simulink model "auv5dof"  (R2021a)
settings: Solver=VariableStepAuto  StartTime=0.0  StopTime=300.00  RelTol=1e-3
settings Model: Creator=aditya-ubuntu  LastModifiedBy=mluser
settings SolverCC: AlgebraicLoopSolver=TrustRegion
settings DataIOCC: ReturnWorkspaceOutputs=off
settings DebuggingCC: SFMachineParentedDataDiag=warning  ArithmeticOperatorsInVariantConditions=warning
settings SFSimCC: CustomCodeUndefinedFunction=UseInterfaceOnly

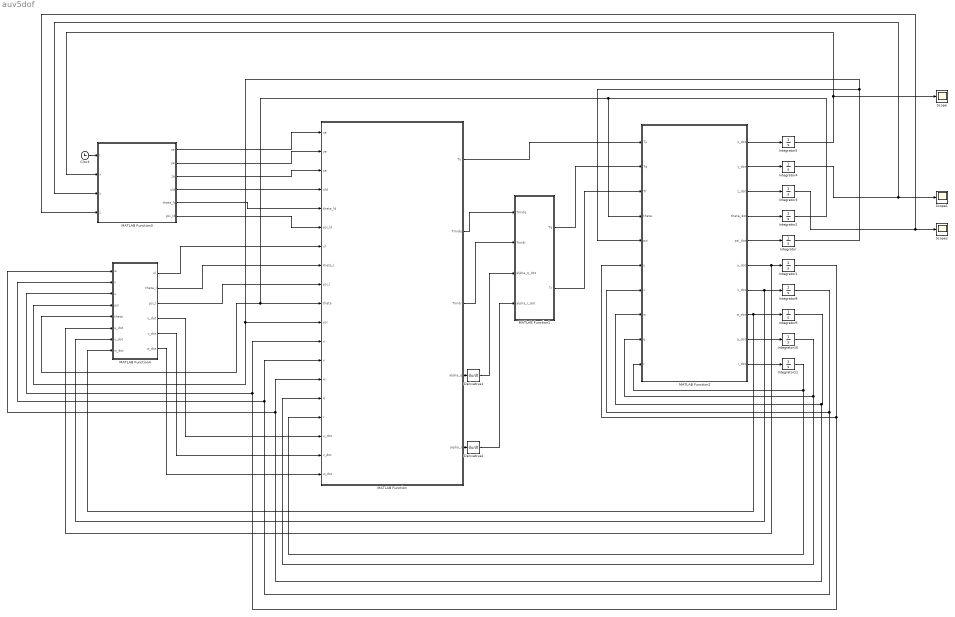
== system auv5dof ==
  Clock : Clock
  Derivative1 : Derivative
  Derivative2 : Derivative
  Integrator{,1..5,8..11} (10 alike) : Integrator
  MATLAB Function : MATLAB Function  TreatAsAtomicUnit=on
  MATLAB Function1 : MATLAB Function  TreatAsAtomicUnit=on
  MATLAB Function2 : MATLAB Function  TreatAsAtomicUnit=on
  MATLAB Function3 : MATLAB Function  TreatAsAtomicUnit=on
  MATLAB Function4 : MATLAB Function  TreatAsAtomicUnit=on
  Scope : Scope
  Scope1 : Scope
  Scope2 : Scope
  wires:
  MATLAB Function2/1(x_dot) -> Integrator5/1
  MATLAB Function2/2(y_dot) -> Integrator4/1
  MATLAB Function2/3(z_dot) -> Integrator3/1
  MATLAB Function2/4(theta_dot) -> Integrator2/1
  MATLAB Function2/5(psi_dot) -> Integrator/1
  MATLAB Function2/6(u_dot) -> MATLAB Function4/6("u_dot "), Integrator1/1
  Integrator5/1 -> Scope/1, MATLAB Function3/2(x)
  Integrator4/1 -> MATLAB Function3/3(y), Scope1/1
  MATLAB Function2/7(v_dot) -> MATLAB Function4/7("v_dot "), Integrator8/1
  MATLAB Function2/8(w_dot) -> MATLAB Function4/8("w_dot "), Integrator9/1
  MATLAB Function2/9(q_dot) -> Integrator10/1
  MATLAB Function2/10(r_dot) -> Integrator11/1
  Integrator10/1 -> MATLAB Function/15(q), MATLAB Function2/9(q)
  Integrator9/1 -> MATLAB Function4/1(w), MATLAB Function/14(w), MATLAB Function2/8(w)
  Integrator8/1 -> MATLAB Function/13(v), MATLAB Function4/2(v), MATLAB Function2/7(v)
  Integrator1/1 -> MATLAB Function/12(u), MATLAB Function4/3(u), MATLAB Function2/6(u)
  Integrator/1 -> MATLAB Function2/5(psi), MATLAB Function4/4(psi), MATLAB Function/11(psi)
  Integrator2/1 -> MATLAB Function4/5(theta), MATLAB Function/10(theta), MATLAB Function2/4(theta)
  Integrator11/1 -> MATLAB Function/16(r), MATLAB Function2/10(r)
  MATLAB Function4/2(theta_l) -> MATLAB Function/8(theta_l)
  MATLAB Function4/3(psi_l) -> MATLAB Function/9(psi_l)
  MATLAB Function4/1(ul) -> MATLAB Function/7(ul)
  MATLAB Function3/1(xe) -> MATLAB Function/1(xe)
  MATLAB Function3/2(ye) -> MATLAB Function/2(ye)
  MATLAB Function3/3(ze) -> MATLAB Function/3(ze)
  MATLAB Function3/4(uld) -> MATLAB Function/4(uld)
  MATLAB Function3/5(theta_ld) -> MATLAB Function/5(theta_ld)
  MATLAB Function3/6(psi_ld) -> MATLAB Function/6(psi_ld)
  Integrator3/1 -> MATLAB Function3/4(z), Scope2/1
  Clock/1 -> MATLAB Function3/1(t)
  MATLAB Function/1(Tu) -> MATLAB Function2/1(Tu)
  MATLAB Function/2(Tmidq) -> MATLAB Function1/1(Tmidq)
  MATLAB Function/3(Tmidr) -> MATLAB Function1/2(Tmidr)
  MATLAB Function/4(alpha_q) -> Derivative1/1
  Derivative1/1 -> MATLAB Function1/3(alpha_q_dot)
  MATLAB Function/5(alpha_r) -> Derivative2/1
  Derivative2/1 -> MATLAB Function1/4(alpha_r_dot)
  MATLAB Function1/1(Tq) -> MATLAB Function2/2(Tq)
  MATLAB Function1/2(Tr) -> MATLAB Function2/3(Tr)
  MATLAB Function4/4(u_dot) -> MATLAB Function/17(u_dot)
  MATLAB Function4/5(v_dot) -> MATLAB Function/18(v_dot)
  MATLAB Function4/6(w_dot) -> MATLAB Function/19(w_dot)

== matlab function auv5dof/MATLAB Function2 ==
  data: x_dot output; y_dot output; z_dot output; theta_dot output; psi_dot output; u_dot output; v_dot output; w_dot output; q_dot output; r_dot output; Tu input; Tq input; Tr input; theta input; psi input; u input; v input; w input; q input; r input
function [ x_dot, y_dot, z_dot, theta_dot, psi_dot, u_dot, v_dot, w_dot, q_dot, r_dot] = outputfn5dof(Tu, Tq, Tr, theta, psi, u, v, w, q, r)
    

    m = [ 1116 2133 2133 36.7 4061 4061];

    onebym = [1/1116 1/2133 1/2133 1/36.7 1/4061 1/4061];
    
    d = [ 25.5 138 138 10 490 490];
    
    row = 1000;
    g = 9.8;
    invtri = 1;
    Gml = 1;
    fu = (m(2)*v*r*onebym(1)) - (m(3)*w*q*onebym(1));
    fv = (-(m(1)*u*r*onebym(2)));
    fw = (m(1)*u*q*onebym(3));
    fq = ((m(3)-m(1))*u*w*onebym(5) - row*g*invtri*Gml*onebym(5)*sin(theta));
    fr = (m(1)-m(2))*u*v*onebym(6);
    
    x_dot = u*cos(theta)*cos(psi) - v*sin(psi) + w*sin(theta)*cos(psi);
    y_dot = u*cos(theta)*sin(psi) + v*cos(psi) + w*sin(theta)*sin(psi);
    z_dot = -u*sin(theta) + w*cos(theta);
    
    theta_dot = q;
    psi_dot = r*sec(theta);
    
    u_dot = fu- onebym(1)*Tu - d(1)*u*onebym(1);
    v_dot = fv - d(2)*onebym(2)*v;
    w_dot = fw - d(3)*onebym(3)*w;
    q_dot = fq + onebym(5)*Tq - d(5)*onebym(5)*q;
    r_dot = fr + onebym(6)*Tr - d(6)*onebym(6)*r; 
    
end

== matlab function auv5dof/MATLAB Function3 ==
  data: xe output; ye output; ze output; uld output; theta_ld output; psi_ld output; t input; x input; y input; z input
function [xe,ye,ze,uld,theta_ld,psi_ld] = fcn(t,x,y,z)
    
    if( t<= 90)
        xd = 0;
        yd = 0;
        zd = 0;
        uld = 1.5;
        theta_ld = 0;
        psi_ld = 0;
    else
        xd = 0;
        yd = 20;
        zd = 0;
        uld = 1.5;
        theta_ld = -10;
        psi_ld = 0.06;
    end
    
    xe = x - xd;
    ye = y - yd;
    ze = z - zd;
end

== matlab function auv5dof/MATLAB Function4 ==
  data: w input; v input; u input; psi input; theta input; ul output; theta_l output; psi_l output; u_dot output; v_dot output; w_dot output; u_dot input; v_dot input; w_dot input
function [ul, theta_l, psi_l, u_dot, v_dot, w_dot] = sphericalfcn(w,v,u,psi,theta, u_dot,v_dot,w_dot)
    
    ul = sqrt(u^2 + v^2 + w^2);
    theta_l = asin((sqrt(u^2+w^2)/ul)*(sin(theta + atan(-w/u))));
    psi_l = psi + atan(u/u*cos(theta));
    
end

== matlab function auv5dof/MATLAB Function1 ==
  data: Tq output; Tr output; Tmidq input; Tmidr input; alpha_q_dot input; alpha_r_dot input
function [Tq, Tr] = fcn(Tmidq, Tmidr, alpha_q_dot, alpha_r_dot)

    m5 = 4061;
    m6 = 4061;
    
    Tq = m5*( Tmidq + alpha_q_dot);
    Tr = m6*( Tmidr + alpha_r_dot);
       
end

== matlab function auv5dof/MATLAB Function ==
  data: Tu output; Tmidq output; Tmidr output; xe input; ye input; ze input; uld input; theta_ld input; psi_ld input; ul input; theta_l input; psi_l input; theta input; psi input; u input; v input; w input; q input; r input; alpha_q output; alpha_r output; u_dot input; v_dot input; w_dot input
function [Tu, Tmidq, Tmidr, alpha_q, alpha_r] = controlinputfn5dof(xe, ye, ze, uld, theta_ld, psi_ld, ul, theta_l, psi_l, theta, psi, u, v, w, q, r, u_dot, v_dot, w_dot)
    
    gamma_R = 0.2;
    gamma_r = 1.2;
    gamma_q = 1.2;
    gamma_u = 1;
    gamma_psi = 0.6;
    gamma_theta = 0.6;
    
    k_psi = 0.5;
    k_theta = 0.5;
    k_R = 0.01;
    k_u = 12;
    k_r = 0.9;
    k_q = 0.9;
    
    onebym_u = 1/1116;
    
    re = sqrt(xe^2 + ye^2 + ze^2);
    
    xe_dot = ul*cos(theta_l)*cos(psi_l) - uld*cos(theta_ld)*cos(psi_ld);
    ye_dot = ul*cos(theta_l)*sin(psi_l) - uld*cos(theta_ld)*sin(psi_ld);
    ze_dot = -ul*sin(theta_l) + uld*sin(theta_ld);
    
    theta_l_D_dot = ( (xe^2 + ye^2)*ze_dot - ze*( xe*xe_dot + ye*ye_dot)) / ( re^2*((xe^2 + ye^2)^0.5));
    psi_l_D_dot = ( xe*ye_dot - ye*xe_dot )/(xe^2+ye^2);
    theta_a = -atan(-w/sqrt(u^2+v^2));
    psi_a = atan(v/u);
    
    theta_b = atan( ze / sqrt(xe^2 + ye^2) );
    theta_le = theta_b - theta_l;
    alpha = theta + atan(-w/u);
    B = sqrt(u^2 + w^2)/ul;
    b_theta = (B*cos(alpha))/sqrt(1 - (B*sin(alpha)^2));
    B_dot = (u*u_dot + w*w_dot)/(ul*ul*B);
    
    F_theta_l = ( B_dot*sin(alpha) + B*cos(alpha)*(u_dot*w - u*w_dot)*(u^2 + w^2) ) / (sqrt(1- ((B*sin(alpha))^2)));
    alpha_q = b_theta^(-1)*( theta_l_D_dot - F_theta_l + (gamma_theta^(-1)*( k_theta*theta_le + ((sin(theta_le/2)^2)/(theta_le/2)))));
    eq = alpha_q - q;

    
    psi_b = atan2(ye,xe);
    psi_le = psi_b - psi_l;
    F_psi_l = ( (u*v_dot - u_dot*v)*cos(theta) + u*v*q*sin(theta) ) / ( (u*cos(theta)^2) + v^2 );
    alpha_r = cos(theta)*( psi_l_D_dot - F_psi_l + gamma_psi^(-1)*( k_psi*psi_le + ((sin(psi_le/2)^2)/(psi_le/2))));
    er = alpha_r - r;

    
    A = cos(theta_l)*cos(theta_b)*(cos(psi_le)-1) + cos(theta_le);
    ulD = uld*A + gamma_R^(-1)*k_R*re;
    A_dot = cos(theta_ld)*( cos(theta_b)*sin(psi_ld - psi_b)*psi_l_D_dot - sin(theta_b)*cos(psi_ld - psi_b)*theta_l_D_dot ) + (sin(theta_ld)*cos(theta_b)*theta_l_D_dot);
    ule = ulD - ul;
    re_dot = uld*A - ul*( cos(theta_l)*cos(theta_b)*cos(psi_le-1) + cos(theta_le));
    ulD_dot = uld*A_dot + gamma_R^(-1)*k_r*re_dot;
    
    Tu = onebym_u^(-1)*sec(theta_a)*sec(psi_a)*( ulD_dot + gamma_u^(-1)*(gamma_R*re + k_u*ule) );
    
    Tmidq = gamma_q*(k_q*eq + gamma_theta*theta_le*b_theta);
    
    Tmidr = gamma_r^(-1)*(k_r*er + r*psi_le*sec(theta));
    
end
